simulink model "MEXFunction_udp_test"  (R2022b)
settings: Solver=ode4  StartTime=0.0  StopTime=1  FixedStep=0.1  RelTol=1e-3
InitFcn:
  | %sl_udp_server_init_cb("127.0.0.1", [12300, 12301, 12302, 12303]);
StopFcn:
  | %sl_udp_server_stop_cb();
undefined symbols (not defined in the file): f
libraries: slrealtimeutilitieslib x4, etargetslib x1, instrumentlib x1, slrealtimeiplib x1
settings Model: SimulationMode=accelerator  Creator=javnson  LastModifiedBy=javnson

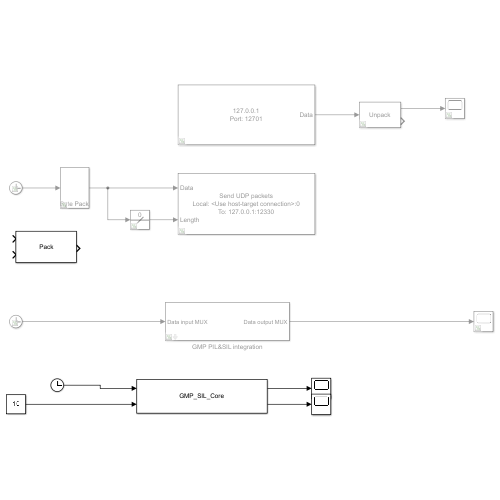
[thumbnail: Simulink's stored preview of the top-level diagram]
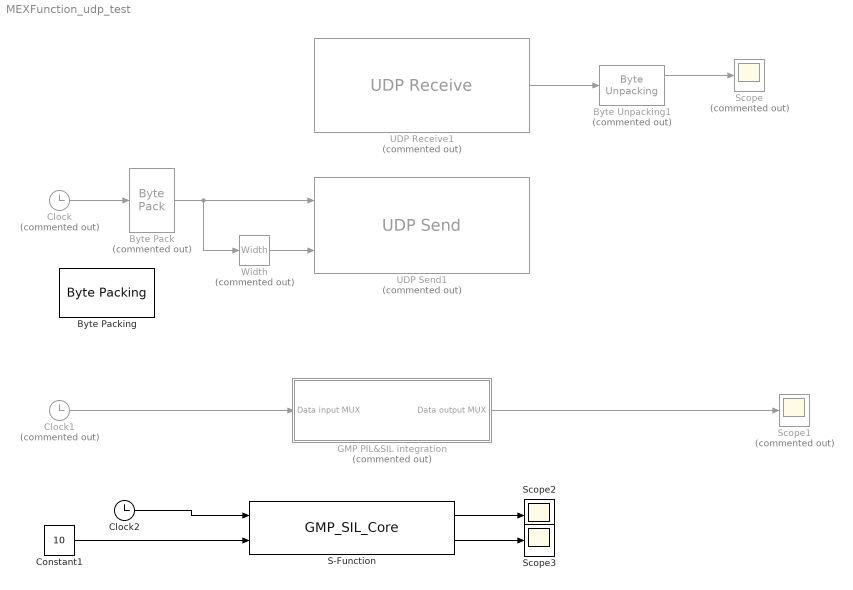
== system MEXFunction_udp_test ==
  Byte Pack : etargetslib/Byte Pack  Commented=on  datatypes={'double'}  byteAlign=1
  Byte Packing : slrealtimeutilitieslib/Byte Packing  MaskPackedDataType=uint8  MaskUnpackedDataTypes={'uint8','uint8'}  MaskAlignment=1
  Byte Unpacking1 : slrealtimeutilitieslib/Byte Unpacking  Commented=on  MaskUnpackedDataTypes={'double','double'}  MaskUnpackedDataSizes={[1],[1]}  MaskAlignment=1
  Clock : Clock  Commented=on
  Clock1 : Clock  Commented=on
  Clock2 : Clock
  Constant1 : Constant  Value=10
  GMP PIL&SIL integration : Subsystem  Commented=on  mask{ByteAlign=1, InputData={'double'}, OutputData={'double'}, OutputDataDim={[1]}, recv_len=8}
      mask init:
      | sl_udp_server_init_cb("127.0.0.1", [12300, 12301, 12302, 12303]);
      mask DialogControl Container4 Prompt: Input&&Output
      mask DialogControl Control2 Prompt: Input Data
      mask DialogControl Control3 Prompt: Output Data
      mask DialogControl Control6 Prompt: Output Data Dimensions
      mask DialogControl Control4 Prompt: Output Data length:
      mask DialogControl Container5 Prompt: Advance
      mask DialogControl Control5 Prompt: Byte Alignment:
  S-Function : S-Function  FunctionName=GMP_SIL_Core  Parameters=NumberUnpackedPorts, UnpackedDataTypes, UnpackedDataSizes, NumberPackedPorts, PackedDataTypes, PackedDataSizes, Alignment  SFunctionDeploymentMode=off  EnableBusSupport=off  mask{MaskPackedDataTypes={'double','double'}, MaskPackedDataSizes={[1],[1]}, MaskUnpackedDataTypes={'double','double'}, MaskUnpackedDataSizes={[1],[1]}, MaskAlignment=1}
      mask init:
      | % MDL invoke parameters
      | % NumberUnpackedPorts, UnpackedDataTypes, UnpackedDataSizes, 
      | % NumberPackedPorts, PackedDataTypes, PackedDataSizes, 
      | % Alignment
      | 
      | % source: MaskUnpackedDataTypes, MaskUnpackedDataSizes
      | % source: MaskPackedDataTypes, MaskUnpackedDataSizes
      | % source: MaskAlignment
      | [NumberUnpackedPorts, UnpackedDataTypes, UnpackedDataSizes, ...
      |      NumberPackedPorts, PackedDataTypes, PackedDataSizes, ...
      |      Alignment] = mdl_gmp_simulink_core( ...
      |      MaskUnpackedDataTypes, MaskUnpackedDataSizes, ...
      |      MaskPackedDataTypes, MaskPackedDataSizes,...
      |      MaskAlignment);
      mask TypeOptions MaskAlignment: 1 | 2 | 4 | 8
      mask DialogControl ParameterGroupVar Prompt: Parameters:
      mask DialogControl Control3 Prompt: Data (sent) types (cell array):(pack)
      mask DialogControl Control7 Prompt: Data (send) port dimisions (cell array) (pack), disabled
      mask DialogControl Control5 Prompt: Data (received) types (cell array):(unpack)
      mask DialogControl Control6 Prompt: Data (received) port dimisions (cell array)(unpacked)
      mask DialogControl Control4 Prompt: Byte Alignment:
  Scope : Scope  Commented=on
  Scope1 : Scope  Commented=on
  Scope2 : Scope
  Scope3 : Scope
  UDP Receive1 : instrumentlib/UDP Receive  Commented=on  LocalAddress=127.0.0.1  LocalPort=12701  EnablePortSharing=off  Host=localhost  Port=12701  GetLatestData=on  DataSize=[ 8 ]  DataType=int8  ASCIIFormatting=%f,  Terminator=LF  CustomTerminator=10  ByteOrder=little-endian  EnableBlockingMode=on  Timeout=15  SampleTime=1e-3  SimulateUsing=Interpreted execution
  UDP Send1 : slrealtimeiplib/UDP Send  Commented=on  useHostTargetConn=on  toAddress='127.0.0.1'  toPort=12330  sampleTime=1e-3  enableMessage=off
  Width : Width  Commented=on
  wires:
  UDP Receive1/1 -> Byte Unpacking1/1
  Byte Unpacking1/1 -> Scope/1
  Byte Pack/1 -> Width/1, UDP Send1/1
  Width/1 -> UDP Send1/2
  Clock/1 -> Byte Pack/1
  Clock1/1 -> GMP PIL&SIL integration/1(Data input MUX)
  GMP PIL&SIL integration/1(Data output MUX) -> Scope1/1
  Clock2/1 -> S-Function/1
  Constant1/1 -> S-Function/2
  S-Function/1 -> Scope2/1
  S-Function/2 -> Scope3/1

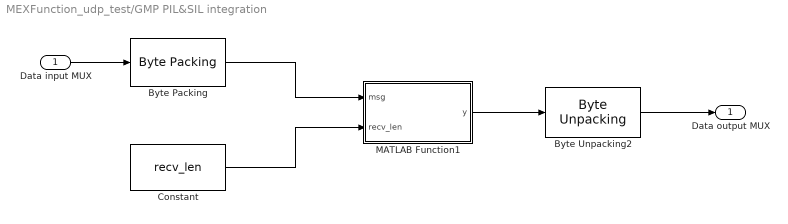
== system MEXFunction_udp_test/GMP PIL&SIL integration ==
  Data input MUX : Inport
  Byte Packing : slrealtimeutilitieslib/Byte Packing  MaskPackedDataType=int8  MaskUnpackedDataTypes=InputData  MaskAlignment=1
  Byte Unpacking2 : slrealtimeutilitieslib/Byte Unpacking  MaskUnpackedDataTypes=OutputData  MaskUnpackedDataSizes=OutputDataDim  MaskAlignment=1
  Constant : Constant  Value=recv_len  LockScale=on
  MATLAB Function1 : MATLAB Function  TreatAsAtomicUnit=on
  Data output MUX : Outport
  wires:
  Data input MUX/1 -> Byte Packing/1
  Byte Packing/1 -> MATLAB Function1/1(msg)
  MATLAB Function1/1(y) -> Byte Unpacking2/1
  Byte Unpacking2/1 -> Data output MUX/1
  Constant/1 -> MATLAB Function1/2(recv_len)

== matlab function MEXFunction_udp_test/GMP PIL&SIL integration/MATLAB Function1 ==
  data: msg input; y output int8 size=1024; recv_len input
function y = fcn(msg,recv_len)

persistent y_tmp

if(isempty(y_tmp))
    y_tmp = zeros(1, 1024,'int8');
end

y_tmp(1,1:recv_len) = udp_recv(recv_len);
udp_send(msg);

y = y_tmp(1,1:recv_len);

end
